simulink model "state_space_delay_2"  (R2018b)
settings: Solver=VariableStepAuto  StartTime=0.0  StopTime=0.5  RelTol=1e-3
values from neighbouring files (symbols this model uses):
  C = K * (k_p + 2 * s)/(1 + s/100) * (s^2 + s + 4)/(1 + s * T)^2    [continous_controller.m]    (also in disturbance_rejection.m = 20 * (10 + 2 * s + 10/s)/(1 + s/100) * (s^2 + s + 4)/(1 + s ; lqr_delay.m = eye(4); pole_placement_delay.m = eye(4))
  K_d = place(sys_discrete.A, sys_discrete.B, discrete_poles)    [pole_placement_delay.m]
  K_delay = place(sys_discrete.A, sys_discrete.B, discrete_poles)    [pole_placement_delay.m]
  selector = [0, 0, 0, 1]    [lqr_delay.m]    (also in pole_placement_delay.m)
  sys_discrete = c2d(sys, 2*pi/sampling_freq, 'zoh')    [control_input_bound.m]    (also in delayed_input.m = (c2d(sys, 2*pi/sampling_freq, 'zoh')); discrete_pole_placement.m = (c2d(sys, 2*pi/sampling_freq, 'zoh')); discretization.m; lqr_controller.m)
undefined symbols (not defined in the file or in its folder): DiscIntNeverNeededParam
settings Model: Creator=lorenzoterenzi  LastModifiedBy=lorenzoterenzi

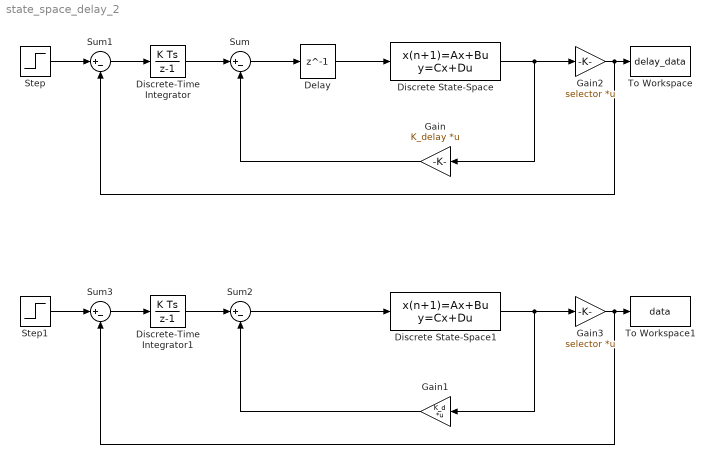
== system state_space_delay_2 ==
  Delay : Delay  DelayLength=1  InitialCondition=0
  Discrete State-Space : DiscreteStateSpace  A=sys_discrete.A  B=sys_discrete.B  C=C  D=[0;0;0;0]  SampleTime=sys_discrete.Ts
  Discrete State-Space1 : DiscreteStateSpace  A=sys_discrete.A  B=sys_discrete.B  C=C  D=[0;0;0;0]  SampleTime=sys_discrete.Ts
  Discrete-Time Integrator : DiscreteIntegrator  gainval=2 * 10^8  SampleTime=-1  ICPrevOutput=DiscIntNeverNeededParam  ICPrevScaledInput=DiscIntNeverNeededParam
  Discrete-Time Integrator1 : DiscreteIntegrator  gainval=10^9  SampleTime=-1  ICPrevOutput=DiscIntNeverNeededParam  ICPrevScaledInput=DiscIntNeverNeededParam
  Gain : Gain  Gain=K_delay  Multiplication=Matrix(K*u)
  Gain1 : Gain  Gain=K_d  Multiplication=Matrix(K*u)
  Gain2 : Gain  Gain=selector  Multiplication=Matrix(K*u)
  Gain3 : Gain  Gain=selector  Multiplication=Matrix(K*u)
  Step : Step  Time=0  SampleTime=0
  Step1 : Step  Time=0  SampleTime=0
  Sum{,1..3} (4 alike) : Sum  Inputs=|+-
  To Workspace : ToWorkspace  VariableName=delay_data  SaveFormat=Timeseries  SampleTime=-1
  To Workspace1 : ToWorkspace  VariableName=data  SaveFormat=Timeseries  SampleTime=-1
  wires:
  Sum/1 -> Delay/1
  Delay/1 -> Discrete State-Space/1
  Discrete State-Space/1 -> Gain2/1, Gain/1
  Gain/1 -> Sum/2
  Gain2/1 -> Sum1/2, To Workspace/1
  Discrete-Time Integrator/1 -> Sum/1
  Sum1/1 -> Discrete-Time Integrator/1
  Step/1 -> Sum1/1
  Gain3/1 -> Sum3/2, To Workspace1/1
  Gain1/1 -> Sum2/2
  Discrete State-Space1/1 -> Gain3/1, Gain1/1
  Step1/1 -> Sum3/1
  Sum2/1 -> Discrete State-Space1/1
  Sum3/1 -> Discrete-Time Integrator1/1
  Discrete-Time Integrator1/1 -> Sum2/1
